simulink model "BACKUP"  (R2023b)
settings: Solver=VariableStepAuto  StartTime=0.0  StopTime=10.0  RelTol=1e-3
values from neighbouring files (symbols this model uses):
  C_PM = 1.758e-3    (= 0.001758)    [HVDCMMCInterconnectionParam.m]
  Carm = C_PM/Nb_PM    (= 4.88333333333e-05)    [HVDCMMCInterconnectionParam.m]
  Cfilter = 1/(Larm*wc2)    (= 4.78421193241e-05)    [HVDCMMCInterconnectionParam.m]
  Cg = 50e-9    (= 5e-08)    [HVDCMMCInterconnectionParam.m]
  Dd11 = Dd(1:nsw,1:nsw);        if(isempty(Dd11)) Dd11 = zeros(3,3); end    [DSS.m]    (also in DSS_test.m)
  Dd12 = Dd(1:nsw,nsw+1:end);    if(isempty(Dd12)) Dd12 = zeros(3,3); end    [DSS.m]    (also in DSS_test.m)
  Fnom = 50    [HVDCMMCInterconnectionParam.m]
  HRM = 2    [HVDCMMCInterconnectionParam.m]
  Ib_ac = (2/3)*Pnom/Vb_ac    [HVDCMMCInterconnectionParam.m]
  Ki_Ireg = 6    [HVDCMMCInterconnectionParam.m]
  Ki_Preg = 1.0    (= 1)    [HVDCMMCInterconnectionParam.m]
  Ki_Qreg = 1.0    (= 1)    [HVDCMMCInterconnectionParam.m]
  Ki_VDCreg = 100    [HVDCMMCInterconnectionParam.m]
  Kp_Ireg = 0.6    [HVDCMMCInterconnectionParam.m]
  Kp_Preg = 0.5/3    (= 0.166666666667)    [HVDCMMCInterconnectionParam.m]
  Kp_Qreg = 0.5/3    (= 0.166666666667)    [HVDCMMCInterconnectionParam.m]
  Kp_VDCreg = 4    [HVDCMMCInterconnectionParam.m]
  L_cable = 15e-3    (= 0.015)    [HVDCMMCInterconnectionParam.m]
  Larm = Larm_pu*(Zb_ac/(2*pi*Fnom))    [HVDCMMCInterconnectionParam.m]
  Lff = Larm_pu/2    (= 0.075)    [HVDCMMCInterconnectionParam.m]
  Limits_Ireg = [ 2.0  -2.0]    [HVDCMMCInterconnectionParam.m]
  Limits_Preg = [ 1.2, 0.8 ]    [HVDCMMCInterconnectionParam.m]
  Limits_Qreg = [ 0.25, -0.25 ]    [HVDCMMCInterconnectionParam.m]
  Limits_VDCreg = [ 2.0  -2.0]    [HVDCMMCInterconnectionParam.m]
  Lxfo = 0.12    [HVDCMMCInterconnectionParam.m]
  Nb_PM = 36    [HVDCMMCInterconnectionParam.m]
  Pnom = 1000e6    (= 1000000000)    [HVDCMMCInterconnectionParam.m]
  R_cable = 0.5    [HVDCMMCInterconnectionParam.m]
  R_startup = 400    [HVDCMMCInterconnectionParam.m]
  Rarm = Rarm_pu*Zb_ac    [HVDCMMCInterconnectionParam.m]
  Rff = Rarm_pu/2    (= 0.00075)    [HVDCMMCInterconnectionParam.m]
  Rfilter = 1/(Cfilter*w)*30    (= 1996.002)    [HVDCMMCInterconnectionParam.m]
  Rg = 100    [HVDCMMCInterconnectionParam.m]
  Rxfo = 0.003    [HVDCMMCInterconnectionParam.m]
  Ts = Ts_Control    (= 4e-05)    [HVDCMMCInterconnectionParam.m]
  Ts_Control = 40e-6    (= 4e-05)    [HVDCMMCInterconnectionParam.m]
  Ts_Power = 20e-6    (= 2e-05)    [HVDCMMCInterconnectionParam.m]
  Vb_ac = sqrt(2/3)*Vnom_sec    [HVDCMMCInterconnectionParam.m]
  Vc0_PM = 0    [HVDCMMCInterconnectionParam.m]
  Vnom_dc = 640e3    (= 640000)    [HVDCMMCInterconnectionParam.m]
  Vnom_prim = 400e3    (= 400000)    [HVDCMMCInterconnectionParam.m]
  Vnom_sec = 333e3    (= 333000)    [HVDCMMCInterconnectionParam.m]
  w = 2*pi*Fnom    (= 314.159265359)    [HVDCMMCInterconnectionParam.m]
  Zb_ac = Vb_ac/Ib_ac    [HVDCMMCInterconnectionParam.m]
undefined symbols (not defined in the file or in its folder): Ad1, Bd1, Cd1, DiscIntNeverNeededParam, gcbh, HrmOrd, Pcc, sps_AC, sps_ACDC, sps_rtmsupport, SYS, Ts_EMT
libraries: spsSeriesRLCBranchLib x22, simulink x20, spsCurrentMeasurementLib x13, spsControlledVoltageSourceLib x12, DQN_Lib x9, spsdq0toabcLib x3, powerlib_extras x3, spsGroundLib x3, spsBreakerLib x3, spsParallelRLCBranchLib x3, eeGeneralControl x2, dspspect3 x2
(part 3 of 5)

== system BACKUP/Discrete State-Space2 ==
  note: Implement discretized state-space model using Tustin or TBE method
      |
      | BE      -> SM.DSSmethod=1
      | Tustin  -> SM.DSSmethod=2
      |
      |
      | Tustin
      | ------
      | Ad = inv(I - Ts/2*A)*(I + Ts/2*A)
      | Bd = inv(I - Ts/2*A)*B
      | Cd = C*inv(I - Ts/2*A)*Ts
      | Dd = C*inv(I - Ts/2*A)*B*Ts/2  + D  =  Cd*B/2
      |
      | TBE
      | ---
      | Ad = inv(I - Ts*A)
      | Bd = inv(I - Ts*A)*B
      | Cd = C*inv(I - Ts*A)*Ts
      | Dd = C*inv(I - Ts*A)*B*Ts  + D  =  Cd*B
      |
      | I = eye(SM.nState,SM.nState)
  U : Inport
  Constant : Constant  Value=Ad1
  Constant1 : Constant  Value=Cd1
  Constant2 : Constant  Value=Bd1
  Constant3 : Constant  Value=Dd1
  Constant5 : Constant  Commented=on  Value=sps_AC.A
  Constant6 : Constant  Commented=on  Value=sps_AC.B
  Constant7 : Constant  Commented=on  Value=sps_AC.C
  Constant8 : Constant  Commented=on  Value=sps_AC.D
  Discretize BE or Tustin : Subsystem  Commented=on  AncestorBlock="DQN_Machines/DQN_Mac_V1/Discretize  BE or Tustin"
  Ihistory_Flux : Subsystem  AncestorBlock=DQN_Machines/DQN_Mac_V1/Ihistory_Flux
  Y : Outport
  wires:
  Constant/1 -> [Ad]
  Constant2/1 -> [Bd]
  Constant1/1 -> [Cd]
  Constant3/1 -> [Dd1]
  Constant7/1 -> Discretize BE or Tustin/3(C)
  Constant6/1 -> Discretize BE or Tustin/2(B)
  Constant8/1 -> Discretize BE or Tustin/4(D)
  Constant5/1 -> Discretize BE or Tustin/1(A)
  U/1 -> Ihistory_Flux/1(u)
  Ihistory_Flux/1(Ihyst) -> Y/1
  [Ad] -> Ihistory_Flux/2(Ad)
  [Bd] -> Ihistory_Flux/3(Bd)
  [Cd] -> Ihistory_Flux/4(Cd)
  [Dd1] -> Ihistory_Flux/5(D)

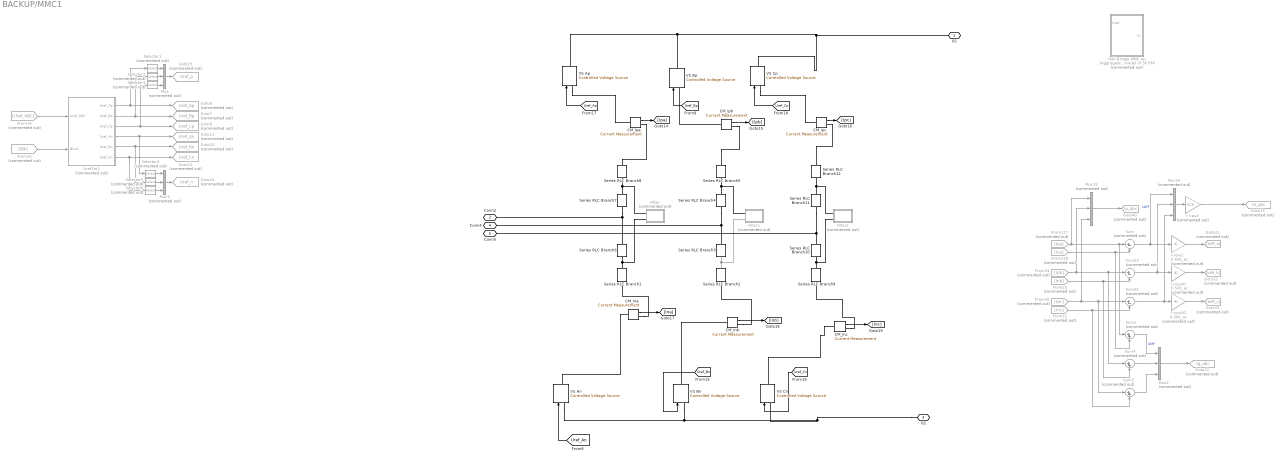
== system BACKUP/MMC1 ==
  CM_Ina : spsCurrentMeasurementLib/Current Measurement  PhasorSimulation=off  OutputType=Complex  PSBequivalent=0
  CM_Inb : spsCurrentMeasurementLib/Current Measurement  PhasorSimulation=off  OutputType=Complex  PSBequivalent=0
  CM_Inc : spsCurrentMeasurementLib/Current Measurement  PhasorSimulation=off  OutputType=Complex  PSBequivalent=0
  CM_Ipa : spsCurrentMeasurementLib/Current Measurement  PhasorSimulation=off  OutputType=Complex  PSBequivalent=0
  CM_Ipb : spsCurrentMeasurementLib/Current Measurement  PhasorSimulation=off  OutputType=Complex  PSBequivalent=0
  CM_Ipc : spsCurrentMeasurementLib/Current Measurement  PhasorSimulation=off  OutputType=Complex  PSBequivalent=0
  Filter : Subsystem  Commented=on
      mask Display: disp('Filter')
  Filter1 : Subsystem  Commented=on
      mask Display: disp('Filter')
  Filter2 : Subsystem  Commented=on
      mask Display: disp('Filter')
  From117 : From  Commented=on  GotoTag=Ipa
  From118 : From  Commented=on  GotoTag=Ina
  From14 : From  Commented=on  GotoTag=Uref_ABC  TagVisibility=global
  From16 : From  Commented=on  GotoTag=Blk  TagVisibility=global
  From20 : From  Commented=on  GotoTag=Ipc
  From22 : From  Commented=on  GotoTag=Inc
  From24 : From  Commented=on  GotoTag=Ipb
  From25 : From  Commented=on  GotoTag=Inb
  Goto10 : Goto  Commented=on  GotoTag=Uref_Bn  TagVisibility=global
  Goto11 : Goto  Commented=on  GotoTag=Uref_An  TagVisibility=global
  Goto12 : Goto  Commented=on  GotoTag=Uref_Cn  TagVisibility=global
  Goto13 : Goto  Commented=on  GotoTag=Id_abc  TagVisibility=global
  Goto22 : Goto  Commented=on  GotoTag=Ig_abc  TagVisibility=global
  Goto23 : Goto  Commented=on  GotoTag=Uref_p  TagVisibility=global
  Goto24 : Goto  Commented=on  GotoTag=Uref_n  TagVisibility=global
  Goto31 : Goto  Commented=on  GotoTag=Idiff_a
  Goto32 : Goto  Commented=on  GotoTag=Idiff_b
  Goto33 : Goto  Commented=on  GotoTag=Idiff_c
  Goto40 : Goto  Commented=on  GotoTag=Ip_abc  TagVisibility=global
  Goto7 : Goto  Commented=on  GotoTag=Uref_Bp  TagVisibility=global
  Goto8 : Goto  Commented=on  GotoTag=Uref_Ap  TagVisibility=global
  Goto9 : Goto  Commented=on  GotoTag=Uref_Cp  TagVisibility=global
  Half-Bridge MMC Ap (Aggregate model of 36 PM) : Subsystem  Commented=on  DialogController=POWERSYS.PowerSysDialog  LoadFcn=sps_rtmsupport('LoadFcn',gcbh);  StartFcn=sps_rtmsupport('StartFcn',gcbh);  StopFcn=sps_rtmsupport('StopFcn',gcbh);  mask(Half-Bridge MMC){ModelType=Aggregate model, n=36, C=C_PM, Vc_Initial=Vc0_PM, Ron=1e-3, Rs=1e6, Cs=inf, Ron_Diode=1e-3, Rs_Diode=1e6, Cs_Diode=inf, Vf_Diode=1e-3, Rs_CurrentSource=inf, Ts=Ts_Power}
      mask prompts: ModelType "Model type:"; n "Number of power modules"; C "Capacitor value (F)"; Vc_Initial "Capacitor initial voltage (V):"; Ron "Device on-state resistance (Ohms)"; Rs "Snubber resistance (Ohms)"; Cs "Snubber capacitance (F)"; Ron_Diode "Diode on-state resistance (Ohms)"; Rs_Diode "Diode snubber resistance (Ohms)"; Cs_Diode "Diode snubber capacitance (F)"; Vf_Diode "Diode forward voltage (V)"; Rs_CurrentSource "Current source snubber resistance (Ohms)"; Ts "Sample time (s):"
      mask help: Implements a half-bridge modular multilevel converter. The converter consists of multiple series-connected power modules. Each power module consists of one half-bridge and one capacitor on the DC side.
      mask init:
      | % block=gcb;
      | % [WantBlockChoice,Index1,MT,SPID] = powericon('FullBridgeMMCInit', block, ModelType, n, Ts, 2);
      | % powericon('SetInternalModels','set',block,WantBlockChoice);
      settings: LibrarySourceBlock=spsHalfBridgeMMCLib/Half-Bridge MMC  CopyFcn=sps_rtmsupport('CopyFcn',gcbh);  DeleteFcn=sps_rtmsupport('DeleteFcn',gcbh);  UndoDeleteFcn=sps_rtmsupport('UndoDeleteFcn',gcbh);  ModelCloseFcn=sps_rtmsupport('ModelCloseFcn',gcbh);  PreSaveFcn=sps_rtmsupport('PreSaveFcn',gcbh);  PostSaveFcn=sps_rtmsupport('PostSaveFcn',gcbh);  NameChangeFcn=sps_rtmsupport('NameChangeFcn',gcbh);  PreCopyFcn=sps_rtmsupport('PreCopyFcn',gcbh);  OpenFcn=sps_rtmsupport('OpenFcn',gcbh, [1]);  CloseFcn=sps_rtmsupport('CloseFcn',gcbh);  PreDeleteFcn=sps_rtmsupport('PreDeleteFcn',gcbh);
      mask Help: helpview(psbhelp);
      mask TypeOptions ModelType: Switching devices | Switching function | Average model (Uref-controlled) | Aggregate model
      mask Callback ModelType: powericon('FullBridgeMMCCback',gcb)
      mask Display:
      | x1=-0.04;
      | plot([0.5 0.80]+x1,[0.95 0.95])
      | plot([0.5 0.5]+x1,[0.95,0.80])
      | plot([0.5 0.38]+x1,[0.80 0.74])
      | plot([0.38 0.38]+x1,[0.80 0.62])
      | plot([0.38 0.5]+x1,[0.68 0.62])
      | plot([0.5 0.5]+x1,[0.62 0.52])
      | plot([0.45 0.5 0.43]+x1,[0.68 0.62 0.60])
      | %
      | y1=0.40;
      | plot([0.5 0.5]+x1,[0.95,0.80]-y1)
      | plot([0.5 0.38]+x1,[0.80 0.74]-y1)
      | plot([0.38 0.38]+x1,[0.80 0.62]-y1)
      | plot([0.38 0.5]+x1,[0.68 0.62]-y1)
      | plot([0.5 0.5]+x1,[0.62 0.52]-y1)
      | plot([0.45 0.5 0.43]+x1,[0.68 0.62 0.60]-y1)
      | plot([0.5 0.5]+x1,[0.2,0.10])
      | plot([0.5 0.80]+x1,[0.1 0.1])
      | %
      | plot([0.5 0.6]+x1,[0.84 0.84])
      | plot([0.6 0.6]+x1,[0.84 0.74])
      | plot([0.6 0.56]+x1,[0.74 0.69])
      | plot([0.6 0.64]+x1,[0.74 0.69])
      | plot([0.56 0.64]+x1,[0.69 0.69])
      | plot([0.6 0.6]+x1,[0.69 0.57])
      | plot([0.5 0.6]+x1,[0.57 0.57])
      | plot([0.55 0.65]+x1,[0.74 0.74])
      | %
      | y2=0.4;
      | plot([0.5 0.6]+x1,[0.84 0.84]-y2)
      | plot([0.6 0.6]+x1,[0.84 0.74]-y2)
      | plot([0.6 0.56]+x1,[0.74 0.69]-y2)
      | plot([0.6 0.64]+x1,[0.74 0.69]-y2)
      | plot([0.56 0.64]+x1,[0.69 0.69]-y2)
      | plot([0.6 0.6]+x1,[0.69 0.57]-y2)
      | plot([0.5 0.6]+x1,[0.57 0.57]-y2)
      | plot([0.55 0.65]+x1,[0.74 0.74]-y2)
      | %
      | plot([0.5 0.23]+x1,[0.5 0.5])
      | plot([0.23 0.23]+x1,[0.5 0.53])
      | plot([0.23 0.23]+x1,[0.55 0.58])
      | plot([0.23 0.23]+x1,[0.61 0.64])
      | %
      | plot([0.5 0.23]+x1,[0.1 0.1])
      | plot([0.23 0.23]+x1,[0.1 0.06])
      | plot([0.23 0.23]+x1,[0.04 0.01])
      | %
      | plot([0.34 0.34]+x1,[0.65 0.75])
      | plot([0.28 0.34]+x1,[0.7 0.7])
      | %
      | plot([0.34 0.34]+x1,[0.65 0.75]-y2)
      | plot([0.28 0.34]+x1,[0.7 0.7]-y2)
      | %
      | % Capacitor
      | plot([0.8 0.8]+x1,[0.51 0.95])
      | plot([0.72 0.88]+x1,[0.51 0.51])
      | plot([0.72 0.88]+x1,[0.51 0.51]-0.04)
      | plot([0.8 0.8]+x1,[0.47 0.1])
      | 
      | color('blue')
      | % switch lower(ModelType)
      | %     case 'average model (uref-controlled)'
      | %         port_label('input',1,'Uref')
      | %     case 'aggregate model'
      | %         port_label('input',1,'Uref')
      | %     otherwise
      | %         port_label('input',1,'Uref')
      | % end
      | port_label('output',1,'m')
  I->pu1 : Gain  Commented=on  Gain=0.5/Ib_ac  SaturateOnIntegerOverflow=on  OutDataTypeStr=Inherit: Same as input  ParamDataTypeStr=Inherit: Same as input
  I->pu3 : Gain  Commented=on  Gain=0.5  SaturateOnIntegerOverflow=on  OutDataTypeStr=Inherit: Same as input  ParamDataTypeStr=Inherit: Same as input
  I->pu40 : Gain  Commented=on  Gain=0.5/Ib_ac  SaturateOnIntegerOverflow=on  OutDataTypeStr=Inherit: Same as input  ParamDataTypeStr=Inherit: Same as input
  I->pu50 : Gain  Commented=on  Gain=0.5/Ib_ac  SaturateOnIntegerOverflow=on  OutDataTypeStr=Inherit: Same as input  ParamDataTypeStr=Inherit: Same as input
  Mux{,2..3,15..16} (5 alike) : Mux  Commented=on  Inputs=3
  Selector{1..6} (6 alike) : Selector  Commented=on  InputPortWidth=2  IndexOptions=Index vector (dialog)  Indices=1  OutputSizes=1
  Series RLC Branch{1..12} (12 alike) : spsSeriesRLCBranchLib/Series RLC Branch  LConnTagsString=__new0  RConnTagsString=__new0  BranchType=RL  Resistance=Rarm/2  Inductance=Larm/2  SetiL0=off  InitialCurrent=0  Capacitance=1e-6  Setx0=off  InitialVoltage=0  Measurements=None
  Sum : Sum  Commented=on  Inputs=|+-
  Sum1 : Sum  Commented=on  Inputs=|++
  Sum23 : Sum  Commented=on  Inputs=|+-
  Sum25 : Sum  Commented=on  Inputs=|+-
  Sum4 : Sum  Commented=on  Inputs=|++
  Sum5 : Sum  Commented=on  Inputs=|++
  Uref2m2 : Subsystem  Commented=on
  VS An : spsControlledVoltageSourceLib/Controlled Voltage Source  Initialize=on  Source_Type=AC  Amplitude=0  Phase=0  Frequency=0  Measurements=None
  VS Ap : spsControlledVoltageSourceLib/Controlled Voltage Source  Initialize=on  Source_Type=AC  Amplitude=0  Phase=0  Frequency=0  Measurements=None
  VS Bn : spsControlledVoltageSourceLib/Controlled Voltage Source  Initialize=on  Source_Type=AC  Amplitude=0  Phase=0  Frequency=0  Measurements=None
  VS Bp : spsControlledVoltageSourceLib/Controlled Voltage Source  Initialize=on  Source_Type=AC  Amplitude=0  Phase=0  Frequency=0  Measurements=None
  VS Cn : spsControlledVoltageSourceLib/Controlled Voltage Source  Initialize=on  Source_Type=AC  Amplitude=0  Phase=0  Frequency=0  Measurements=None
  VS Cp : spsControlledVoltageSourceLib/Controlled Voltage Source  Initialize=on  Source_Type=AC  Amplitude=0  Phase=0  Frequency=0  Measurements=None
  O1 : PMIOPort  Side=Right
  Conn2 : PMIOPort  Port=2  Side=Left
  O2 : PMIOPort  Port=3  Side=Right
  Conn4 : PMIOPort  Port=4  Side=Left
  Conn5 : PMIOPort  Port=5  Side=Left
  wires:
  [Uref_An] -> VS An/1
  [Uref_Cp] -> VS Cp/1
  [Uref_Cn] -> VS Cn/1
  CM_Ipb/1 -> [Ipb]
  [Uref_Bn] -> VS Bn/1
  CM_Ina/1 -> [Ina]
  CM_Ipa/1 -> [Ipa]
  CM_Ipc/1 -> [Ipc]
  [Uref_Bp] -> VS Bp/1
  CM_Inc/1 -> [Inc]
  CM_Inb/1 -> [Inb]
  [Uref_Ap] -> VS Ap/1
  Sum4/1 -> Mux2/2
  From117/1 -> Mux15/1, Sum1/1, Sum/1
  Mux16/1 -> I->pu3/1
  From118/1 -> Sum1/2, Sum/2
  Sum25/1 -> Mux16/3, I->pu50/1
  From24/1 -> Mux15/2, Sum4/1, Sum23/1
  Mux15/1 -> Goto40/1
  From25/1 -> Sum4/2, Sum23/2
  Sum1/1 -> Mux2/1  "Idiff"
  I->pu1/1 -> Goto31/1
  I->pu40/1 -> Goto32/1
  Sum/1 -> Mux16/1, I->pu1/1  "Idiff"
  From22/1 -> Sum5/2, Sum25/2
  Sum23/1 -> Mux16/2, I->pu40/1
  I->pu3/1 -> Goto13/1
  From20/1 -> Mux15/3, Sum5/1, Sum25/1
  I->pu50/1 -> Goto33/1
  Sum5/1 -> Mux2/3
  Mux2/1 -> Goto22/1
  Mux3/1 -> Goto24/1
  Selector5/1 -> Mux3/2
  Selector6/1 -> Mux3/3
  Selector3/1 -> Mux/3
  Selector4/1 -> Mux3/1
  Mux/1 -> Goto23/1
  Uref2m2/5(Uref_Bn) -> Selector5/1, Goto10/1
  From14/1 -> Uref2m2/1(Uref_ABC)
  From16/1 -> Uref2m2/2(Block)
  Uref2m2/4(Uref_An) -> Selector4/1, Goto11/1
  Uref2m2/3(Uref_Cp) -> Goto9/1, Selector3/1
  Selector1/1 -> Mux/1
  Uref2m2/6(Uref_Cn) -> Selector6/1, Goto12/1
  Selector2/1 -> Mux/2
  Uref2m2/1(Uref_Ap) -> Selector1/1, Goto8/1
  Uref2m2/2(Uref_Bp) -> Selector2/1, Goto7/1
  connections:
  VS Cp/LConn1 -- CM_Ipc/LConn1
  Series RLC Branch4/LConn1 -- Filter1/LConn1 -- Series RLC Branch5/RConn1
  CM_Ina/RConn1 -- Series RLC Branch1/RConn1
  VS Cp/RConn1 -- O1/RConn1 -- VS Ap/RConn1 -- VS Bp/RConn1
  CM_Ipb/LConn1 -- VS Bp/LConn1
  Series RLC Branch7/LConn1 -- Filter/LConn1 -- Series RLC Branch8/RConn1
  CM_Ipc/RConn1 -- Series RLC Branch12/LConn1
  Series RLC Branch10/RConn1 -- Filter2/LConn2 -- Series RLC Branch9/LConn1
  O2/RConn1 -- VS Cn/LConn1 -- VS Bn/LConn1 -- VS An/LConn1
  Filter1/LConn2 -- Series RLC Branch2/LConn1 -- Series RLC Branch3/RConn1
  VS Ap/LConn1 -- CM_Ipa/LConn1
  VS Bn/RConn1 -- CM_Inb/LConn1
  CM_Inc/RConn1 -- Series RLC Branch9/RConn1
  Series RLC Branch1/LConn1 -- Filter/LConn2 -- Series RLC Branch6/RConn1
  Series RLC Branch12/RConn1 -- Series RLC Branch11/LConn1 -- Filter2/LConn1
  CM_Inb/RConn1 -- Series RLC Branch2/RConn1
  CM_Ipa/RConn1 -- Series RLC Branch8/LConn1
  Series RLC Branch7/RConn1 -- Conn2/RConn1 -- Series RLC Branch6/LConn1
  VS Cn/RConn1 -- CM_Inc/LConn1
  CM_Ipb/RConn1 -- Series RLC Branch5/LConn1
  Series RLC Branch4/RConn1 -- Conn4/RConn1 -- Series RLC Branch3/LConn1
  VS An/RConn1 -- CM_Ina/LConn1
  Series RLC Branch11/RConn1 -- Conn5/RConn1 -- Series RLC Branch10/LConn1

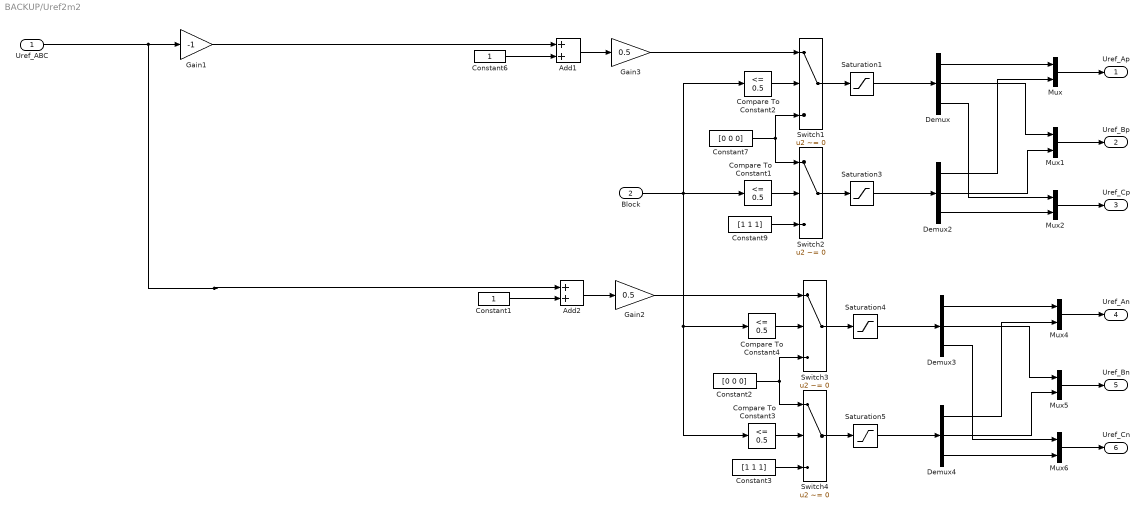
== system BACKUP/Uref2m2 ==
  Uref_ABC : Inport  PortDimensions=3
  Block : Inport  Port=2
  Add1 : Sum
  Add2 : Sum
  Compare To Constant{1..4} (4 alike) : simulink/Logic and Bit Operations/Compare To Constant  relop=<=  const=0.5  OutDataTypeStr=boolean
  Constant1 : Constant
  Constant2 : Constant  Value=[0 0 0]
  Constant3 : Constant  Value=[1 1 1]
  Constant6 : Constant
  Constant7 : Constant  Value=[0 0 0]
  Constant9 : Constant  Value=[1 1 1]
  Demux{,2..4} (4 alike) : Demux  Outputs=3
  Gain1 : Gain  Gain=-1
  Gain2 : Gain  Gain=0.5
  Gain3 : Gain  Gain=0.5
  Mux{,1..2,4..6} (6 alike) : Mux  Inputs=2
  Saturation{1,3..5} (4 alike) : Saturate  UpperLimit=1  LowerLimit=0
  Switch{1..4} (4 alike) : Switch  Criteria=u2 ~= 0  SaturateOnIntegerOverflow=off  InputSameDT=off
  Uref_Ap : Outport
  Uref_Bp : Outport  Port=2
  Uref_Cp : Outport  Port=3
  Uref_An : Outport  Port=4
  Uref_Bn : Outport  Port=5
  Uref_Cn : Outport  Port=6
  wires:
  Add1/1 -> Gain3/1
  Gain3/1 -> Switch1/1
  Constant7/1 -> Switch1/3, Switch2/1
  Compare To Constant1/1 -> Switch2/2
  Constant6/1 -> Add1/2
  Constant9/1 -> Switch2/3
  Compare To Constant2/1 -> Switch1/2
  Gain1/1 -> Add1/1
  Mux/1 -> Uref_Ap/1
  Switch1/1 -> Saturation1/1
  Switch2/1 -> Saturation3/1
  Demux/1 -> Mux/1
  Demux2/1 -> Mux/2
  Demux/2 -> Mux1/1
  Demux2/2 -> Mux1/2
  Demux2/3 -> Mux2/2
  Demux/3 -> Mux2/1
  Demux4/1 -> Mux4/2
  Demux4/2 -> Mux5/2
  Constant1/1 -> Add2/2
  Compare To Constant4/1 -> Switch3/2
  Compare To Constant3/1 -> Switch4/2
  Add2/1 -> Gain2/1
  Constant2/1 -> Switch3/3, Switch4/1
  Block/1 -> Compare To Constant1/1, Compare To Constant4/1, Compare To Constant3/1, Compare To Constant2/1
  Uref_ABC/1 -> Add2/1, Gain1/1
  Switch3/1 -> Saturation4/1
  Demux3/2 -> Mux5/1
  Demux3/3 -> Mux6/1
  Constant3/1 -> Switch4/3
  Demux3/1 -> Mux4/1
  Switch4/1 -> Saturation5/1
  Gain2/1 -> Switch3/1
  Demux4/3 -> Mux6/2
  Saturation1/1 -> Demux/1
  Saturation3/1 -> Demux2/1
  Saturation4/1 -> Demux3/1
  Saturation5/1 -> Demux4/1
  Mux1/1 -> Uref_Bp/1
  Mux2/1 -> Uref_Cp/1
  Mux4/1 -> Uref_An/1
  Mux5/1 -> Uref_Bn/1
  Mux6/1 -> Uref_Cn/1

== system BACKUP/VSRC ==
  In1 : Inport
  Demux9 : Demux  Outputs=3
  Ground : spsGroundLib/Ground  LConnTagsString=a
  VSRC_a : spsControlledVoltageSourceLib/Controlled Voltage Source  Initialize=on  Source_Type=AC  Amplitude=0  Phase=0  Frequency=0  Measurements=None
  VSRC_b : spsControlledVoltageSourceLib/Controlled Voltage Source  Initialize=on  Source_Type=AC  Amplitude=0  Phase=0  Frequency=0  Measurements=None
  VSRC_c : spsControlledVoltageSourceLib/Controlled Voltage Source  Initialize=on  Source_Type=AC  Amplitude=0  Phase=0  Frequency=0  Measurements=None
  a : PMIOPort  Side=Right
  b : PMIOPort  Port=2  Side=Right
  c : PMIOPort  Port=3  Side=Right
  wires:
  In1/1 -> Demux9/1
  Demux9/1 -> VSRC_a/1
  Demux9/2 -> VSRC_b/1
  Demux9/3 -> VSRC_c/1
  connections:
  Ground/LConn1 -- VSRC_b/LConn1 -- VSRC_a/LConn1 -- VSRC_c/LConn1
  VSRC_c/RConn1 -- c/RConn1
  VSRC_b/RConn1 -- b/RConn1
  VSRC_a/RConn1 -- a/RConn1

== system BACKUP/3ph SM/Delay ==
  In1 : Inport
  Gain9 : Gain  Gain=2
  Sum6 : Sum  Inputs=+-  InputSameDT=on  SaturateOnIntegerOverflow=on  OutDataTypeStr=Inherit: Same as first input
  Unit Delay5 : UnitDelay  SampleTime=Ts_Power  HasFrameUpgradeWarning=on
  Unit Delay6 : UnitDelay  SampleTime=Ts_Power  HasFrameUpgradeWarning=on
  Vc : Outport
  wires:
  Unit Delay5/1 -> Sum6/2
  Sum6/1 -> Vc/1  "Vc"
  Unit Delay6/1 -> Gain9/1, Unit Delay5/1
  Gain9/1 -> Sum6/1
  In1/1 -> Unit Delay6/1

== system BACKUP/3ph SM/I_Uref Mult ==
  Uref : Inport
  I : Inport  Port=2
  Demux1 : Demux  Outputs=3
  Demux4 : Demux  Outputs=3
  Mux : Mux  Inputs=3
  Product10 : Product
  Product11 : Product
  Product3 : Product
  Selector : Selector  InputPortWidth=6  IndexOptions=Index vector (dialog)  Indices=[1 4 2 5 3 6]  OutputSizes=1
  Sum1 : Sum  Inputs=1  InputSameDT=on  SaturateOnIntegerOverflow=on  OutDataTypeStr=Inherit: Same as first input
  Sum2 : Sum  Inputs=1  InputSameDT=on  SaturateOnIntegerOverflow=on  OutDataTypeStr=Inherit: Same as first input
  Sum3 : Sum  Inputs=1  InputSameDT=on  SaturateOnIntegerOverflow=on  OutDataTypeStr=Inherit: Same as first input
  Out1 : Outport
  wires:
  Sum1/1 -> Mux/2
  Product10/1 -> Sum1/1
  Demux4/3 -> Product11/2
  Demux4/2 -> Product10/2
  Demux4/1 -> Product3/2
  Demux1/1 -> Product3/1
  Demux1/3 -> Product11/1
  Sum3/1 -> Mux/1
  Product11/1 -> Sum2/1
  Product3/1 -> Sum3/1
  Selector/1 -> Demux4/1
  Sum2/1 -> Mux/3
  I/1 -> Selector/1
  Demux1/2 -> Product10/1
  Uref/1 -> Demux1/1
  Mux/1 -> Out1/1

== system BACKUP/3ph SM/MinSum ==
  In1 : Inport
  VoutA : Inport  Port=2
  Demux : Demux  Outputs=3
  Demux1 : Demux  Outputs=3
  Min1 : MinMax  Inputs=2
  Min2 : MinMax  Inputs=2
  Min4 : MinMax  Inputs=2
  Mux27 : Mux  Inputs=3
  Sum of Elements1 : Sum  Inputs=+
  Sum of Elements2 : Sum  Inputs=+
  Sum of Elements3 : Sum  Inputs=+
  Out1 : Outport
  wires:
  Min2/1 -> Sum of Elements3/1
  Demux/3 -> Min2/1
  Min1/1 -> Sum of Elements2/1
  Demux/1 -> Min4/1
  Min4/1 -> Sum of Elements1/1  "min"
  Demux1/2 -> Min1/2
  Demux1/1 -> Min4/2
  Mux27/1 -> Out1/1
  Sum of Elements2/1 -> Mux27/2
  VoutA/1 -> Demux1/1
  Sum of Elements3/1 -> Mux27/3
  Demux/2 -> Min1/1
  In1/1 -> Demux/1
  Demux1/3 -> Min2/2
  Sum of Elements1/1 -> Mux27/1

== system BACKUP/3ph SM/Uref_Vc Mult ==
  Uref : Inport
  VcA : Inport  Port=2
  Demux : Demux  Outputs=3
  Demux1 : Demux  Outputs=2
  Demux2 : Demux  Outputs=2
  Demux3 : Demux  Outputs=2
  Demux4 : Demux  Outputs=3
  Mux : Mux  Inputs=3
  Mux1 : Mux  Inputs=2
  Mux2 : Mux  Inputs=2
  Mux4 : Mux  Inputs=2
  Product{1..5,7} (6 alike) : Product
  VoutA : Outport
  wires:
  Demux4/1 -> Product7/2, Product4/2
  Mux4/1 -> Mux/1
  Product4/1 -> Mux4/1  "Vin"
  Demux1/2 -> Product7/1
  Demux1/1 -> Product4/1
  Product7/1 -> Mux4/2  "Vbl"
  Demux/1 -> Demux1/1
  Demux4/2 -> Product2/2, Product1/2
  Product1/1 -> Mux1/1  "Vin"
  Demux2/1 -> Product1/1
  Demux/2 -> Demux2/1
  Demux2/2 -> Product2/1
  Mux1/1 -> Mux/2
  Product2/1 -> Mux1/2  "Vbl"
  Demux4/3 -> Product5/2, Product3/2
  Product3/1 -> Mux2/1  "Vin"
  Demux3/1 -> Product3/1
  Demux/3 -> Demux3/1
  Demux3/2 -> Product5/1
  Mux2/1 -> Mux/3
  Product5/1 -> Mux2/2  "Vbl"
  Uref/1 -> Demux/1
  VcA/1 -> Demux4/1
  Mux/1 -> VoutA/1

== system BACKUP/3ph SM1/Delay ==
  In1 : Inport
  Gain9 : Gain  Gain=2
  Sum6 : Sum  Inputs=+-  InputSameDT=on  SaturateOnIntegerOverflow=on  OutDataTypeStr=Inherit: Same as first input
  Unit Delay5 : UnitDelay  SampleTime=Ts_Power  HasFrameUpgradeWarning=on
  Unit Delay6 : UnitDelay  SampleTime=Ts_Power  HasFrameUpgradeWarning=on
  Vc : Outport
  wires:
  Unit Delay5/1 -> Sum6/2
  Sum6/1 -> Vc/1  "Vc"
  Unit Delay6/1 -> Gain9/1, Unit Delay5/1
  Gain9/1 -> Sum6/1
  In1/1 -> Unit Delay6/1

== system BACKUP/3ph SM1/I_Uref Mult ==
  Uref : Inport
  I : Inport  Port=2
  Demux1 : Demux  Outputs=3
  Demux4 : Demux  Outputs=3
  Mux : Mux  Inputs=3
  Product10 : Product
  Product11 : Product
  Product3 : Product
  Selector : Selector  InputPortWidth=6  IndexOptions=Index vector (dialog)  Indices=[1 4 2 5 3 6]  OutputSizes=1
  Sum1 : Sum  Inputs=1  InputSameDT=on  SaturateOnIntegerOverflow=on  OutDataTypeStr=Inherit: Same as first input
  Sum2 : Sum  Inputs=1  InputSameDT=on  SaturateOnIntegerOverflow=on  OutDataTypeStr=Inherit: Same as first input
  Sum3 : Sum  Inputs=1  InputSameDT=on  SaturateOnIntegerOverflow=on  OutDataTypeStr=Inherit: Same as first input
  Out1 : Outport
  wires:
  Sum1/1 -> Mux/2
  Product10/1 -> Sum1/1
  Demux4/3 -> Product11/2
  Demux4/2 -> Product10/2
  Demux4/1 -> Product3/2
  Demux1/1 -> Product3/1
  Demux1/3 -> Product11/1
  Sum3/1 -> Mux/1
  Product11/1 -> Sum2/1
  Product3/1 -> Sum3/1
  Selector/1 -> Demux4/1
  Sum2/1 -> Mux/3
  I/1 -> Selector/1
  Demux1/2 -> Product10/1
  Uref/1 -> Demux1/1
  Mux/1 -> Out1/1

== system BACKUP/3ph SM1/MinSum ==
  In1 : Inport
  VoutA : Inport  Port=2
  Demux : Demux  Outputs=3
  Demux1 : Demux  Outputs=3
  Min1 : MinMax  Inputs=2
  Min2 : MinMax  Inputs=2
  Min4 : MinMax  Inputs=2
  Mux27 : Mux  Inputs=3
  Sum of Elements1 : Sum  Inputs=+
  Sum of Elements2 : Sum  Inputs=+
  Sum of Elements3 : Sum  Inputs=+
  Out1 : Outport
  wires:
  Min2/1 -> Sum of Elements3/1
  Demux/3 -> Min2/1
  Min1/1 -> Sum of Elements2/1
  Demux/1 -> Min4/1
  Min4/1 -> Sum of Elements1/1  "min"
  Demux1/2 -> Min1/2
  Demux1/1 -> Min4/2
  Mux27/1 -> Out1/1
  Sum of Elements2/1 -> Mux27/2
  VoutA/1 -> Demux1/1
  Sum of Elements3/1 -> Mux27/3
  Demux/2 -> Min1/1
  In1/1 -> Demux/1
  Demux1/3 -> Min2/2
  Sum of Elements1/1 -> Mux27/1

== system BACKUP/3ph SM1/Uref_Vc Mult ==
  Uref : Inport
  VcA : Inport  Port=2
  Demux : Demux  Outputs=3
  Demux1 : Demux  Outputs=2
  Demux2 : Demux  Outputs=2
  Demux3 : Demux  Outputs=2
  Demux4 : Demux  Outputs=3
  Mux : Mux  Inputs=3
  Mux1 : Mux  Inputs=2
  Mux2 : Mux  Inputs=2
  Mux4 : Mux  Inputs=2
  Product{1..5,7} (6 alike) : Product
  VoutA : Outport
  wires:
  Demux4/1 -> Product7/2, Product4/2
  Mux4/1 -> Mux/1
  Product4/1 -> Mux4/1  "Vin"
  Demux1/2 -> Product7/1
  Demux1/1 -> Product4/1
  Product7/1 -> Mux4/2  "Vbl"
  Demux/1 -> Demux1/1
  Demux4/2 -> Product2/2, Product1/2
  Product1/1 -> Mux1/1  "Vin"
  Demux2/1 -> Product1/1
  Demux/2 -> Demux2/1
  Demux2/2 -> Product2/1
  Mux1/1 -> Mux/2
  Product2/1 -> Mux1/2  "Vbl"
  Demux4/3 -> Product5/2, Product3/2
  Product3/1 -> Mux2/1  "Vin"
  Demux3/1 -> Product3/1
  Demux/3 -> Demux3/1
  Demux3/2 -> Product5/1
  Mux2/1 -> Mux/3
  Product5/1 -> Mux2/2  "Vbl"
  Uref/1 -> Demux/1
  VcA/1 -> Demux4/1
  Mux/1 -> VoutA/1

== system BACKUP/BAK/3ph SM1 ==
  Vconv (3ph) : Inport
  Vref (3ph) : Inport  Port=2
  Iarm (3ph) : Inport  Port=3
  Constant1 : Constant  Value=Vb_ac
  Delay : Subsystem
  Discrete-Time Integrator1 : DiscreteIntegrator  IntegratorMethod=Integration: Trapezoidal  gainval=1  SampleTime=Ts_Power  UpperSaturationLimit=5000  LowerSaturationLimit=500  ICPrevOutput=DiscIntNeverNeededParam  ICPrevScaledInput=DiscIntNeverNeededParam
  Gain16 : Gain  Gain=Nb_PM
  Gain8 : Gain  Gain=1/(C_PM*Nb_PM)
  I_Uref Mult : Subsystem
  MinSum : Subsystem
  Mux2 : Mux  Inputs=2
  Saturation2 : Saturate  UpperLimit=inf  LowerLimit=0
  Subtract1 : Sum  Inputs=+-
  Unit Delay1 : UnitDelay  SampleTime=Ts_Power  HasFrameUpgradeWarning=on
  Uref_Vc Mult : Subsystem
  Varm (3ph) : Outport
  wires:
  Subtract1/1 -> MinSum/1(In1)
  Vconv (3ph)/1 -> Subtract1/2
  Constant1/1 -> Subtract1/1
  Vref (3ph)/1 -> Gain16/1
  MinSum/1(Out1) -> Varm (3ph)/1
  Gain8/1 -> Discrete-Time Integrator1/1
  Discrete-Time Integrator1/1 -> Delay/1(In1)
  Delay/1(Vc) -> Uref_Vc Mult/2(VcA)
  Gain16/1 -> I_Uref Mult/1(Uref), Uref_Vc Mult/1(Uref)
  Saturation2/1 -> Mux2/2
  Iarm (3ph)/1 -> Saturation2/1, Mux2/1
  Mux2/1 -> Unit Delay1/1
  Unit Delay1/1 -> I_Uref Mult/2(I)
  I_Uref Mult/1(Out1) -> Gain8/1
  Uref_Vc Mult/1(VoutA) -> MinSum/2(VoutA)

== system BACKUP/BAK/Delay3 ==
  In1 : Inport
  Gain9 : Gain  Gain=2
  Sum6 : Sum  Inputs=+-  InputSameDT=on  SaturateOnIntegerOverflow=on  OutDataTypeStr=Inherit: Same as first input
  Unit Delay5 : UnitDelay  SampleTime=Ts_Power  HasFrameUpgradeWarning=on
  Unit Delay6 : UnitDelay  SampleTime=Ts_Power  HasFrameUpgradeWarning=on
  Vc : Outport
  wires:
  Unit Delay5/1 -> Sum6/2
  Sum6/1 -> Vc/1  "Vc"
  Unit Delay6/1 -> Gain9/1, Unit Delay5/1
  Gain9/1 -> Sum6/1
  In1/1 -> Unit Delay6/1

== system BACKUP/BAK/Demux_DQNc_Mat ==

== system BACKUP/BAK/Discrete State-Space ==
  note: Implement discretized state-space model using Tustin or TBE method
      |
      | BE      -> SM.DSSmethod=1
      | Tustin  -> SM.DSSmethod=2
      |
      |
      | Tustin
      | ------
      | Ad = inv(I - Ts/2*A)*(I + Ts/2*A)
      | Bd = inv(I - Ts/2*A)*B
      | Cd = C*inv(I - Ts/2*A)*Ts
      | Dd = C*inv(I - Ts/2*A)*B*Ts/2  + D  =  Cd*B/2
      |
      | TBE
      | ---
      | Ad = inv(I - Ts*A)
      | Bd = inv(I - Ts*A)*B
      | Cd = C*inv(I - Ts*A)*Ts
      | Dd = C*inv(I - Ts*A)*B*Ts  + D  =  Cd*B
      |
      | I = eye(SM.nState,SM.nState)
  U : Inport
  Add : Sum
  Add3 : Sum
  Add4 : Sum  Inputs=+++
  Constant : Constant  Value=Ad1
  Constant1 : Constant  Value=Cd1
  Constant2 : Constant  Value=Bd1
  Constant3 : Constant  Value=Dd11
  Constant4 : Constant  Value=Dd12
  Delay : Delay  DelayLength=1  SampleTime=dt
  Product{5..8,13} (5 alike) : Product  Multiplication=Matrix(*)  SaturateOnIntegerOverflow=on  OutDataTypeStr=Inherit: Same as first input
  Unit Delay2 : UnitDelay  InitialCondition=InitVec  SampleTime=dt  HasFrameUpgradeWarning=on
  Y : Outport
  wires:
  Add3/1 -> Unit Delay2/1
  Delay/1 -> Add/2, Product5/2
  [Cd] -> Product6/1
  Unit Delay2/1 -> Product6/2, Product7/2  "xd"
  Product6/1 -> Add4/1
  Add/1 -> Product13/2
  Product7/1 -> Add3/2  "Ad*X"
  Product13/1 -> Add3/1  "Bd*U"
  [Bd] -> Product13/1
  U/1 -> Delay/1, Product8/2, Add/1
  [Dd1] -> Product8/1
  [Ad] -> Product7/1
  Product8/1 -> Add4/2
  Product5/1 -> Add4/3
  [Dd2] -> Product5/1
  Add4/1 -> Y/1  "Vabc_DQN"
  Constant/1 -> [Ad]
  Constant2/1 -> [Bd]
  Constant1/1 -> [Cd]
  Constant3/1 -> [Dd1]
  Constant4/1 -> [Dd2]

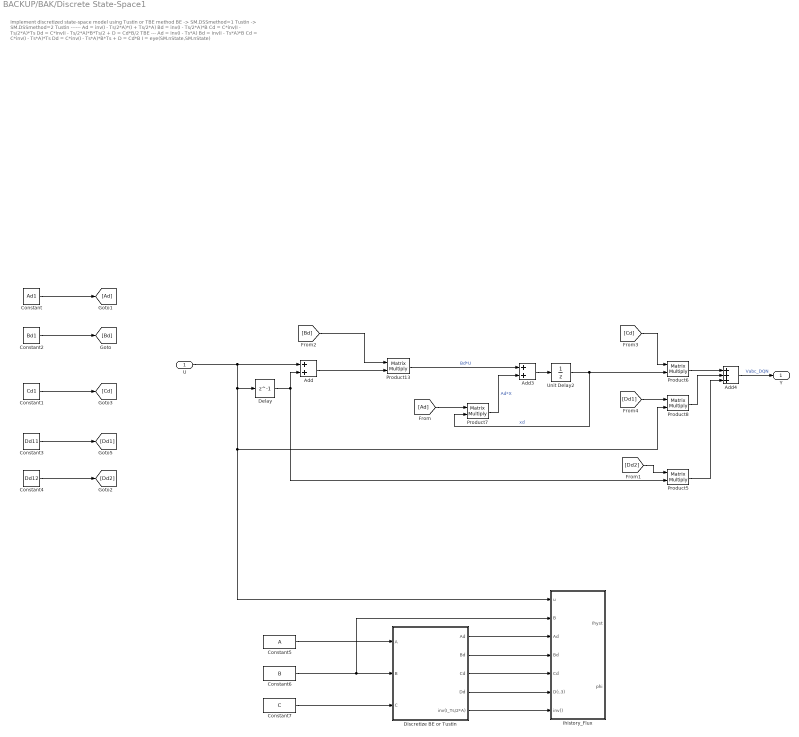
== system BACKUP/BAK/Discrete State-Space1 ==
  note: Implement discretized state-space model using Tustin or TBE method
      |
      | BE      -> SM.DSSmethod=1
      | Tustin  -> SM.DSSmethod=2
      |
      |
      | Tustin
      | ------
      | Ad = inv(I - Ts/2*A)*(I + Ts/2*A)
      | Bd = inv(I - Ts/2*A)*B
      | Cd = C*inv(I - Ts/2*A)*Ts
      | Dd = C*inv(I - Ts/2*A)*B*Ts/2  + D  =  Cd*B/2
      |
      | TBE
      | ---
      | Ad = inv(I - Ts*A)
      | Bd = inv(I - Ts*A)*B
      | Cd = C*inv(I - Ts*A)*Ts
      | Dd = C*inv(I - Ts*A)*B*Ts  + D  =  Cd*B
      |
      | I = eye(SM.nState,SM.nState)
  U : Inport
  Add : Sum
  Add3 : Sum
  Add4 : Sum  Inputs=+++
  Constant : Constant  Value=Ad1
  Constant1 : Constant  Value=Cd1
  Constant2 : Constant  Value=Bd1
  Constant3 : Constant  Value=Dd11
  Constant4 : Constant  Value=Dd12
  Constant5 : Constant  Value=A
  Constant6 : Constant  Value=B
  Constant7 : Constant  Value=C
  Delay : Delay  DelayLength=1  SampleTime=Ts
  Discretize BE or Tustin : Subsystem  AncestorBlock="DQN_Machines/DQN_Mac_V1/Discretize  BE or Tustin"
  Ihistory_Flux : Subsystem  AncestorBlock=DQN_Machines/DQN_Mac_V1/Ihistory_Flux
  Product{5..8,13} (5 alike) : Product  Multiplication=Matrix(*)  SaturateOnIntegerOverflow=on  OutDataTypeStr=Inherit: Same as first input
  Unit Delay2 : UnitDelay  InitialCondition=InitVec  SampleTime=dt  HasFrameUpgradeWarning=on
  Y : Outport
  wires:
  Constant4/1 -> [Dd2]
  Constant3/1 -> [Dd1]
  Constant1/1 -> [Cd]
  Constant2/1 -> [Bd]
  Constant/1 -> [Ad]
  [Dd2] -> Product5/1
  Product5/1 -> Add4/3
  Product8/1 -> Add4/2
  [Ad] -> Product7/1
  [Dd1] -> Product8/1
  U/1 -> Add/1, Ihistory_Flux/1(u), Product8/2, Delay/1
  [Bd] -> Product13/1
  Product13/1 -> Add3/1  "Bd*U"
  Product7/1 -> Add3/2  "Ad*X"
  Add/1 -> Product13/2
  Product6/1 -> Add4/1
  Unit Delay2/1 -> Product7/2, Product6/2  "xd"
  [Cd] -> Product6/1
  Delay/1 -> Product5/2, Add/2
  Add3/1 -> Unit Delay2/1
  Discretize BE or Tustin/5(inv(I_Ts/2*A)) -> Ihistory_Flux/7(inv())
  Discretize BE or Tustin/2(Bd) -> Ihistory_Flux/4(Bd)
  Constant7/1 -> Discretize BE or Tustin/3(C)
  Constant6/1 -> Ihistory_Flux/2(B), Discretize BE or Tustin/2(B)
  Discretize BE or Tustin/3(Cd) -> Ihistory_Flux/5(Cd)
  Constant5/1 -> Discretize BE or Tustin/1(A)
  Discretize BE or Tustin/1(Ad) -> Ihistory_Flux/3(Ad)
  Discretize BE or Tustin/4(Dd) -> Ihistory_Flux/6(D(:,3))
  Add4/1 -> Y/1  "Vabc_DQN"

== system BACKUP/BAK/Discrete State-Space2 ==
  note: Implement discretized state-space model using Tustin or TBE method
      |
      | BE      -> SM.DSSmethod=1
      | Tustin  -> SM.DSSmethod=2
      |
      |
      | Tustin
      | ------
      | Ad = inv(I - Ts/2*A)*(I + Ts/2*A)
      | Bd = inv(I - Ts/2*A)*B
      | Cd = C*inv(I - Ts/2*A)*Ts
      | Dd = C*inv(I - Ts/2*A)*B*Ts/2  + D  =  Cd*B/2
      |
      | TBE
      | ---
      | Ad = inv(I - Ts*A)
      | Bd = inv(I - Ts*A)*B
      | Cd = C*inv(I - Ts*A)*Ts
      | Dd = C*inv(I - Ts*A)*B*Ts  + D  =  Cd*B
      |
      | I = eye(SM.nState,SM.nState)
  U : Inport
  Add1 : Sum
  Add2 : Sum
  Constant : Constant  Value=Adc
  Constant1 : Constant  Value=Cdc
  Constant2 : Constant  Value=Bdc
  Constant3 : Constant  Value=Ddc
  Delay1 : Delay  DelayLength=1  InitialCondition=InitVec_c  SampleTime=dt
  Gain1 : Gain  Gain=exp(-1i*Ws*dt)
  Product{1..4} (4 alike) : Product  Multiplication=Matrix(*)  SaturateOnIntegerOverflow=on  OutDataTypeStr=Inherit: Same as first input
  Y : Outport
  wires:
  Constant3/1 -> [Dd1]
  Constant1/1 -> [Cd]
  Constant2/1 -> [Bd]
  Constant/1 -> [Ad]
  Product1/1 -> Add1/1  "Bd*U"
  Product2/1 -> Add2/1
  [Dd1] -> Product4/1
  Product4/1 -> Add2/2
  [Bd] -> Product1/1  "u"
  Product3/1 -> Add1/2  "Ad*X"
  [Cd] -> Product2/1
  Delay1/1 -> Gain1/1  "xd"
  Add1/1 -> Delay1/1
  [Ad] -> Product3/1
  U/1 -> Product4/2, Product1/2  "u"
  Gain1/1 -> Product3/2, Product2/2  "xd"
  Add2/1 -> Y/1

== system BACKUP/BAK/Discrete State-Space4 ==
  note: Implement discretized state-space model using Tustin or TBE method
      |
      | BE      -> SM.DSSmethod=1
      | Tustin  -> SM.DSSmethod=2
      |
      |
      | Tustin
      | ------
      | Ad = inv(I - Ts/2*A)*(I + Ts/2*A)
      | Bd = inv(I - Ts/2*A)*B
      | Cd = C*inv(I - Ts/2*A)*Ts
      | Dd = C*inv(I - Ts/2*A)*B*Ts/2  + D  =  Cd*B/2
      |
      | TBE
      | ---
      | Ad = inv(I - Ts*A)
      | Bd = inv(I - Ts*A)*B
      | Cd = C*inv(I - Ts*A)*Ts
      | Dd = C*inv(I - Ts*A)*B*Ts  + D  =  Cd*B
      |
      | I = eye(SM.nState,SM.nState)
  U : Inport
  Constant : Constant  Value=Ad1
  Constant1 : Constant  Value=Cd1
  Constant2 : Constant  Value=Bd1
  Constant3 : Constant  Value=Dd1
  Constant5 : Constant  Commented=on  Value=sps_AC.A
  Constant6 : Constant  Commented=on  Value=sps_AC.B
  Constant7 : Constant  Commented=on  Value=sps_AC.C
  Constant8 : Constant  Commented=on  Value=sps_AC.D
  Discretize BE or Tustin : Subsystem  Commented=on  AncestorBlock="DQN_Machines/DQN_Mac_V1/Discretize  BE or Tustin"
  Ihistory_Flux : Subsystem  AncestorBlock=DQN_Machines/DQN_Mac_V1/Ihistory_Flux
  Y : Outport
  wires:
  [Dd1] -> Ihistory_Flux/5(D)
  [Cd] -> Ihistory_Flux/4(Cd)
  [Bd] -> Ihistory_Flux/3(Bd)
  [Ad] -> Ihistory_Flux/2(Ad)
  U/1 -> Ihistory_Flux/1(u)
  Constant5/1 -> Discretize BE or Tustin/1(A)
  Constant8/1 -> Discretize BE or Tustin/4(D)
  Constant6/1 -> Discretize BE or Tustin/2(B)
  Constant7/1 -> Discretize BE or Tustin/3(C)
  Constant3/1 -> [Dd1]
  Constant1/1 -> [Cd]
  Constant2/1 -> [Bd]
  Constant/1 -> [Ad]
  Ihistory_Flux/1(Ihyst) -> Y/1

== system BACKUP/BAK/Discrete State-Space5 ==
  note: Implement discretized state-space model using Tustin or TBE method
      |
      | BE      -> SM.DSSmethod=1
      | Tustin  -> SM.DSSmethod=2
      |
      |
      | Tustin
      | ------
      | Ad = inv(I - Ts/2*A)*(I + Ts/2*A)
      | Bd = inv(I - Ts/2*A)*B
      | Cd = C*inv(I - Ts/2*A)*Ts
      | Dd = C*inv(I - Ts/2*A)*B*Ts/2  + D  =  Cd*B/2
      |
      | TBE
      | ---
      | Ad = inv(I - Ts*A)
      | Bd = inv(I - Ts*A)*B
      | Cd = C*inv(I - Ts*A)*Ts
      | Dd = C*inv(I - Ts*A)*B*Ts  + D  =  Cd*B
      |
      | I = eye(SM.nState,SM.nState)
  U : Inport
  Constant : Constant  Value=Ad1
  Constant1 : Constant  Value=Cd1
  Constant2 : Constant  Value=Bd1
  Constant3 : Constant  Value=Dd1
  Constant5 : Constant  Commented=on  Value=sps_AC.A
  Constant6 : Constant  Commented=on  Value=sps_AC.B
  Constant7 : Constant  Commented=on  Value=sps_AC.C
  Constant8 : Constant  Commented=on  Value=sps_AC.D
  Discretize BE or Tustin : Subsystem  Commented=on  AncestorBlock="DQN_Machines/DQN_Mac_V1/Discretize  BE or Tustin"
  Ihistory_Flux : Subsystem  AncestorBlock=DQN_Machines/DQN_Mac_V1/Ihistory_Flux
  Y : Outport
  wires:
  Constant/1 -> [Ad]
  Constant2/1 -> [Bd]
  Constant1/1 -> [Cd]
  Constant3/1 -> [Dd1]
  Constant7/1 -> Discretize BE or Tustin/3(C)
  Constant6/1 -> Discretize BE or Tustin/2(B)
  Constant8/1 -> Discretize BE or Tustin/4(D)
  Constant5/1 -> Discretize BE or Tustin/1(A)
  U/1 -> Ihistory_Flux/1(u)
  Ihistory_Flux/1(Ihyst) -> Y/1
  [Ad] -> Ihistory_Flux/2(Ad)
  [Bd] -> Ihistory_Flux/3(Bd)
  [Cd] -> Ihistory_Flux/4(Cd)
  [Dd1] -> Ihistory_Flux/5(D)

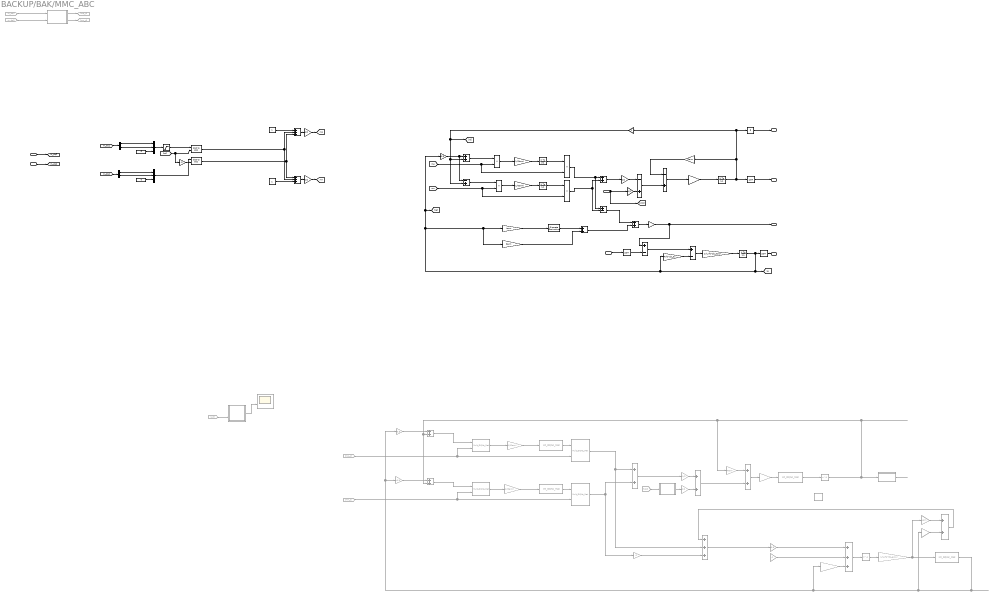
== system BACKUP/BAK/MMC_ABC ==
  m_dq1 : Inport
  m_dq2 : Inport  Port=2
  Vdc : Inport  Port=3
  Vsec : Inport  Port=4
  Add1 : Sum  Inputs=+-
  Add10 : Sum  Commented=on  Inputs=+++
  Add{2,4,7,11,13..14} (6 alike) : Sum  Commented=on
  Add12 : Sum  Commented=on  Inputs=+++
  Add{3,5,8..9} (4 alike) : Sum
  Add6 : Sum  Inputs=-+
  Constant1 : Constant  Value=0
  Constant6 : Constant  Value=0
  Constant74 : Constant
  Constant75 : Constant
  DQn->ABC1 : MATLAB Function  Commented=on  TreatAsAtomicUnit=on  SystemSampleTime=Ts  mask{N=HrmOrd}
      mask prompts: N "Harmonic order:"
  Delay2 : Delay  Commented=on  DelayLength=1  SampleTime=Ts
  Delay3 : Delay  Commented=on  DelayLength=1  SampleTime=Ts
  Demux10 : Demux  Outputs=2
  Demux11 : Demux  Outputs=2
  Discrete Derivative : simulink/Discrete/Discrete Derivative  gainval=1.0  ICPrevScaledInput=0.0  OutMin=[]  OutMax=[]  OutDataType=fixdt(1, 16)  OutScaling=2^-10  DoSatur=off
  Discrete-Time Integrator{,1..3} (4 alike) : DiscreteIntegrator  SampleTime=Ts_Power  ICPrevOutput=DiscIntNeverNeededParam  ICPrevScaledInput=DiscIntNeverNeededParam
  From1 : From  Commented=on  GotoTag=m_dq1  TagVisibility=global
  From2 : From  Commented=on  GotoTag=m_dq2  TagVisibility=global
  From30 : From  Commented=on  GotoTag=wt  TagVisibility=global
  From5 : From  Commented=on  GotoTag=Vdc
  From7 : From  Commented=on  GotoTag=mp_c
  From8 : From  Commented=on  GotoTag=mn_c
  Gain : Gain
  Gain1 : Gain  Gain=0.5
  Gain10 : Gain  Commented=on  Gain=-Rarm
  Gain11 : Gain  Commented=on  Gain=-0.5
  Gain12 : Gain  Gain=-0.5
  Gain13 : Gain  Commented=on  Gain=Rarm
  Gain14 : Gain  Commented=on  Gain=-0.5
  Gain15 : Gain  Commented=on  Gain=1/(Lxfo*Zb_ac/w)
  Gain16 : Gain  Commented=on  Gain=-Rxfo*Zb_ac
  Gain17 : Gain  Commented=on  Gain=-1
  Gain18 : Gain  Commented=on  Gain=1/(Larm)
  Gain2 : Gain  Gain=1/(Carm)
  Gain21 : Gain  Gain=1/(Carm)
  Gain27 : Gain  Gain=1/(Larm)
  Gain28 : Gain  Gain=Rarm
  Gain3 : Gain  Gain=Rarm
  Gain4 : Gain  Commented=on  Gain=Larm
  Gain5 : Gain  Commented=on  Gain=0.5
  Gain6 : Gain  Gain=Larm
  Gain60 : Gain  Gain=1/(Lxfo*Zb_ac/w)
  Gain61 : Gain  Gain=Rxfo*Zb_ac
  Gain7 : Gain  Gain=-2
  Gain8 : Gain  Commented=on  Gain=1/(Carm)
  Gain9 : Gain  Commented=on  Gain=1/(Carm)
  Goto : Goto  Commented=on  GotoTag=mp_c
  Goto3 : Goto  Commented=on  GotoTag=mn_c
  I->pu1 : Gain  Commented=on  Gain=-1/2  SaturateOnIntegerOverflow=on  OutDataTypeStr=Inherit: Same as input  ParamDataTypeStr=Inherit: Same as input
  I->pu{5,12,22,28} (4 alike) : Gain  Gain=1/2  SaturateOnIntegerOverflow=on  OutDataTypeStr=Inherit: Same as input  ParamDataTypeStr=Inherit: Same as input
  I->pu2 : Gain  Commented=on  Gain=-1  SaturateOnIntegerOverflow=on  OutDataTypeStr=Inherit: Same as input  ParamDataTypeStr=Inherit: Same as input
  I->pu3 : Gain  Commented=on  Gain=1/2  SaturateOnIntegerOverflow=on  OutDataTypeStr=Inherit: Same as input  ParamDataTypeStr=Inherit: Same as input
  Int_DQNc_Mat{1..3,5} (4 alike) : DQN_Lib/Int_DQNc_Mat  Commented=on  N=HrmOrd  dt=Ts  w=Ws  InitInt=0*[0.8; 0.6; -0.33]  swFeed=off  R=1  iL=1
  MATLAB Function : MATLAB Function  Commented=on  TreatAsAtomicUnit=on
  MATLAB Function1 : MATLAB Function  Commented=on  TreatAsAtomicUnit=on  mask{N=HrmOrd}
      mask prompts: N "Harmonic order:"
  MATLAB Function2 : MATLAB Function  Commented=on  TreatAsAtomicUnit=on  mask{N=HrmOrd}
      mask prompts: N "Harmonic order:"
  Mult_DQNc_Mat{1..3,5} (4 alike) : DQN_Lib/Mult_DQNc_Mat  Commented=on  N=HrmOrd  HrmDbl=off
  Mux1 : Mux  Inputs=3
  Mux4 : Mux  Inputs=3
  Product{4,6..8} (4 alike) : Product
  SS_DelayPrediction : DQN_Lib/SS_DelayPrediction  Commented=on  N=HrmOrd  Ts=Ts  x0=zeros(3,1)
  Saturation : Saturate  UpperLimit=Limits_Ireg(1)  LowerLimit=Limits_Ireg(2)
  Scope : Scope  Commented=on  NumInputPorts=2
  Subtract2 : Sum  Inputs=+-+
  Subtract5 : Sum  Inputs=+++
  Subtract6 : Sum  Inputs=+-
  Subtract7 : Sum  Inputs=+-
  Sum of Elements : Sum  Inputs=+
  Sum2 : Sum  Inputs=-+  InputSameDT=on  SaturateOnIntegerOverflow=on  OutDataTypeStr=Inherit: Same as first input
  Sum3 : Sum  Inputs=-+  InputSameDT=on  SaturateOnIntegerOverflow=on  OutDataTypeStr=Inherit: Same as first input
  Zero-Order Hold2 : ZeroOrderHold  SampleTime=Ts_Power
  Zero-Order Hold4 : ZeroOrderHold  SampleTime=Ts
  Zero-Order Hold5 : ZeroOrderHold  SampleTime=Ts
  dq0 to abc : spsdq0toabcLib/dq0 to abc  Alignment=90 degrees behind phase A axis
  dq0 to abc1 : spsdq0toabcLib/dq0 to abc  Alignment=90 degrees behind phase A axis
  Vconv : Outport
  Idc : Outport  Port=2
  Id : Outport  Port=3
  Iconv1 : Outport  Port=4  VectorParamsAs1DForOutWhenUnconnected=off
  tag scope: Ig=global, m_dq1=global, m_dq2=global, mn=global, mp=global
  wires:
  Gain21/1 -> Discrete-Time Integrator1/1  "dVn_M"
  Add6/1 -> Product7/1
  Discrete-Time Integrator2/1 -> Zero-Order Hold4/1, Gain/1, Sum of Elements/1, Gain28/1  "dVp_M"
  Gain1/1 -> Add6/1, Add3/1
  Sum2/1 -> Sum3/2
  Add1/1 -> Add8/1
  Add3/1 -> Product4/1  "prod"
  Gain3/1 -> Add5/2  "dVp_M"
  Discrete-Time Integrator1/1 -> Product8/1  "Vn_M"
  Gain6/1 -> Discrete Derivative/1  "dVp_M"
  Discrete Derivative/1 -> Add5/1
  Gain28/1 -> Sum3/1
  Product8/1 -> Add9/2, Add1/2
  Add9/1 -> I->pu5/1  "dVp_M"
  Product7/1 -> Gain21/1
  Discrete-Time Integrator/1 -> Product6/1  "Vp_M"
  Add8/1 -> Gain12/1
  Gain2/1 -> Discrete-Time Integrator/1  "dVp_M"
  I->pu12/1 -> Sum2/2
  I->pu5/1 -> Sum2/1
  Sum3/1 -> Gain27/1
  Gain12/1 -> Vconv/1, Subtract6/1  "prod"
  Add5/1 -> Add8/2
  Sum of Elements/1 -> Idc/1
  m_dq1/1 -> [m_dq1]
  m_dq2/1 -> [m_dq2]
  Gain/1 -> [Id], Add6/2, Add3/2
  Gain27/1 -> Discrete-Time Integrator2/1
  Subtract7/1 -> Gain60/1
  Vsec/1 -> Zero-Order Hold2/1
  Gain61/1 -> Subtract7/2
  Subtract6/1 -> Subtract7/1
  Gain60/1 -> Discrete-Time Integrator3/1
  Discrete-Time Integrator3/1 -> Zero-Order Hold5/1, [Ig], Gain1/1, Gain3/1, Gain6/1, Gain61/1, [Ig]  "Igd"
  I->pu22/1 -> [mp]
  Constant75/1 -> Subtract5/3
  Subtract2/1 -> I->pu22/1
  Constant74/1 -> Subtract2/1
  [m_dq2] -> Demux11/1
  [m_dq1] -> Demux10/1
  Demux10/2 -> Mux4/2
  Gain7/1 -> dq0 to abc1/2
  I->pu28/1 -> [mn]
  Demux10/1 -> Mux4/1
  Mux1/1 -> dq0 to abc1/1
  Constant6/1 -> Mux4/3
  Mux4/1 -> Saturation/1
  Demux11/2 -> Mux1/2
  Subtract5/1 -> I->pu28/1
  [wt] -> Gain7/1, dq0 to abc/2
  Saturation/1 -> dq0 to abc/1
  Demux11/1 -> Mux1/1
  Constant1/1 -> Mux1/3
  [mp] -> Product6/2, Product4/2
  [mn] -> Product8/2, Product7/2
  dq0 to abc/1 -> Subtract5/2, Subtract2/2
  dq0 to abc1/1 -> Subtract5/1, Subtract2/3
  Zero-Order Hold2/1 -> Subtract6/2
  Vdc/1 -> I->pu12/1, [Vdc]
  Zero-Order Hold4/1 -> Id/1
  Zero-Order Hold5/1 -> Iconv1/1
  Product6/1 -> Add1/1, Add9/1  "Iabc_B22 (A)"
  Product4/1 -> Gain2/1
  Gain14/1 -> Add12/1
  Gain17/1 -> Add10/3
  Add13/1 -> Add10/1
  Mult_DQNc_Mat5/1 -> Add2/1, Add10/2
  Add11/1 -> Add14/2
  Mult_DQNc_Mat2/1 -> Gain8/1
  Gain4/1 -> Add13/1  "dVp_M"
  Gain9/1 -> Int_DQNc_Mat2/1
  I->pu2/1 -> Add12/2
  From1/1 -> MATLAB Function1/1(m1_dq)
  From8/1 -> Mult_DQNc_Mat3/2, Mult_DQNc_Mat1/2
  ? -> I->pu2/1
  Gain16/1 -> Add12/3
  I->pu1/1 -> Add11/1
  Add10/1 -> Gain14/1
  Mult_DQNc_Mat1/1 -> Gain9/1
  MATLAB Function/1(y) -> ?
  Mult_DQNc_Mat3/1 -> Gain17/1, Add2/2
  Gain10/1 -> Add14/1
  Gain18/1 -> Int_DQNc_Mat3/1
  Gain15/1 -> Int_DQNc_Mat5/1, Gain4/1
  Add7/1 -> Mult_DQNc_Mat2/1
  Add14/1 -> Gain18/1
  MATLAB Function2/1(Vdc_c) -> I->pu3/1
  Delay3/1 -> Gain15/1
  Int_DQNc_Mat3/1 -> Delay2/1  "dw"
  Gain8/1 -> Int_DQNc_Mat1/1
  Add2/1 -> I->pu1/1
  Int_DQNc_Mat5/1 -> Gain5/1, Gain11/1, Gain16/1, Gain13/1
  Add12/1 -> Delay3/1
  From7/1 -> Mult_DQNc_Mat5/2, Mult_DQNc_Mat2/2
  Int_DQNc_Mat1/1 -> Mult_DQNc_Mat5/1
  Gain11/1 -> Add4/1
  MATLAB Function1/1(mp_c) -> Goto/1
  Gain13/1 -> Add13/2
  Gain5/1 -> Add7/1
  I->pu3/1 -> Add11/2
  MATLAB Function1/2(mn_c) -> Goto3/1
  From2/1 -> MATLAB Function1/2(m2_dq)
  Add4/1 -> Mult_DQNc_Mat1/1
  Int_DQNc_Mat2/1 -> Mult_DQNc_Mat3/1
  From5/1 -> MATLAB Function2/1(Vdc)
  Delay2/1 -> MATLAB Function/1(u), Add4/2, Add7/2, Gain10/1
  From30/1 -> DQn->ABC1/2(tho)
  DQn->ABC1/1(Xabc) -> Scope/2

== system BACKUP/BAK/Mux_DQNc_Mat ==
  In1 : Inport
  In2 : Inport  Port=2
  In3 : Inport  Port=3
  In4 : Inport  Port=4
  Mux : Concatenate  NumInputs=4  Mode=Multidimensional array
  Out1 : Outport
  wires:
  In1/1 -> Mux/1
  In2/1 -> Mux/2
  In3/1 -> Mux/3
  In4/1 -> Mux/4
  Mux/1 -> Out1/1

== system BACKUP/BAK/SS_DQNc_Mat_Dicrete ==
  note: Implement discretized state-space model using Tustin or TBE method
      |
      | BE      -> SM.DSSmethod=1
      | Tustin  -> SM.DSSmethod=2
      |
      |
      | Tustin
      | ------
      | Ad = inv(I - Ts/2*A)*(I + Ts/2*A)
      | Bd = inv(I - Ts/2*A)*B
      | Cd = C*inv(I - Ts/2*A)*Ts
      | Dd = C*inv(I - Ts/2*A)*B*Ts/2  + D  =  Cd*B/2
      |
      | TBE
      | ---
      | Ad = inv(I - Ts*A)
      | Bd = inv(I - Ts*A)*B
      | Cd = C*inv(I - Ts*A)*Ts
      | Dd = C*inv(I - Ts*A)*B*Ts  + D  =  Cd*B
      |
      | I = eye(SM.nState,SM.nState)
  U : Inport
  Add : Sum
  Add1 : Sum
  Add2 : Sum
  Add3 : Sum  Commented=on
  Add4 : Sum  Commented=on
  Constant1 : Constant  Commented=on  Value=Cd
  Constant2 : Constant  Commented=on  Value=Dd
  Constant3 : Constant  Value=Ad
  Constant4 : Constant  Value=Bd
  Constant5 : Constant  Value=Cd
  Constant6 : Constant  Value=Dd
  Constant7 : Constant  Commented=on  Value=Bd
  Constant8 : Constant  Commented=on  Value=Ad
  Delay1 : Delay  Commented=on  DelayLength=1  SampleTime=dt
  Gain : Gain  Commented=on  Gain=exp(-1i*Ws*dt)
  Gain1 : Gain  Gain=0.5
  Gain2 : Gain  Commented=on  Gain=exp(-1i*Ws*dt)
  Product{1..2,5,7} (4 alike) : Product  Commented=on  Multiplication=Matrix(*)  SaturateOnIntegerOverflow=on  OutDataTypeStr=Inherit: Same as first input
  Product{9..12} (4 alike) : Product  Multiplication=Matrix(*)  SaturateOnIntegerOverflow=on  OutDataTypeStr=Inherit: Same as first input
  Unit Delay1 : UnitDelay  InitialCondition=InitVec  SampleTime=dt  HasFrameUpgradeWarning=on
  Unit Delay2 : UnitDelay  SampleTime=dt  HasFrameUpgradeWarning=on
  Y : Outport
  wires:
  Constant2/1 -> Product7/1
  Product7/1 -> Add4/2
  U/1 -> Add/1, Unit Delay2/1, Product1/2, Product7/2  "u"
  Add3/1 -> Delay1/1
  Product1/1 -> Add3/1  "Bd*U"
  Constant7/1 -> Product1/1  "u"
  Constant1/1 -> Product2/1
  Product2/1 -> Add4/1
  Product5/1 -> Add3/2  "Ad*X"
  Constant8/1 -> Product5/1  "Ad*X"
  Delay1/1 -> Product2/2, Product5/2  "xd"
  Constant5/1 -> Product10/1
  Add/1 -> Gain1/1
  Unit Delay2/1 -> Add/2
  Constant4/1 -> Product9/1
  Gain1/1 -> Product9/2, Product12/2
  Product11/1 -> Add1/2  "Ad*X"
  Add1/1 -> Unit Delay1/1
  Product9/1 -> Add1/1  "Bd*U"
  Unit Delay1/1 -> Product10/2, Product11/2  "xd"
  Product10/1 -> Add2/1
  Constant6/1 -> Product12/1
  Constant3/1 -> Product11/1
  Product12/1 -> Add2/2
  Add2/1 -> Y/1  "Vabc_DQN"

== system BACKUP/BAK/SW1 ==
  note: (Uref)
  Blk : Inport
  Uref_1ph : Inport  Port=2
  Add1 : Sum  Inputs=+-
  Add3 : Sum  Inputs=-+
  Compare To Constant1 : simulink/Logic and Bit Operations/Compare To Constant  relop=<=  const=0.5  OutDataTypeStr=boolean
  Constant1 : Constant  Value=ones(1,1)
  Constant4 : Constant  Value=ones(1,1)
  Data Type Conversion2 : DataTypeConversion  OutDataTypeStr=double  SaturateOnIntegerOverflow=off  RndMeth=Floor
  Gain4 : Gain  Gain=0.5
  Mux1 : Mux  Inputs=2
  Product1 : Product
  Product5 : Product
  Saturation : Saturate  UpperLimit=1  LowerLimit=-1
  Out1 : Outport
  wires:
  Uref_1ph/1 -> Saturation/1
  Constant4/1 -> Add1/1
  Gain4/1 -> Add1/2, Product5/2
  Mux1/1 -> Out1/1
  Data Type Conversion2/1 -> Product5/1, Product1/1
  Compare To Constant1/1 -> Data Type Conversion2/1
  Saturation/1 -> Add3/1
  Add3/1 -> Gain4/1
  Add1/1 -> Product1/2
  Product5/1 -> Mux1/2
  Constant1/1 -> Add3/2
  Product1/1 -> Mux1/1
  Blk/1 -> Compare To Constant1/1
